simulink library "SUB_ECU_L4_MABX_HW_Interface_PIC_PB"  (R2018a)
settings: Solver=VariableStepAuto  StartTime=0.0  StopTime=10.0  RelTol=1e-3
PostLoadFcn:
  | , if any(exist('dsrtsu_mdlpostloadfcn', 'file') == [2, 3, 6]), try dsrtsu_mdlpostloadfcn('Execute', bdroot); catch fprintf('Error in PostLoadFcn (dsrtsu_mdlpostloadfcn) for model "%s":\n %s\n', bdroot, lasterr); end, end,
undefined symbols (not defined in the file or in its folder): CANR_PROPB_REAX_3_13_CHANNEL_APV, CANR_PROPB_REAX_4_13_CHANNEL_APV, CANR_PROPB_XPR_1_50_CHANNEL_APV, ENUM_CAN_RX_T, ENUM_CAN_TX_T, ENUM_REAX_OPERATION_MODE_T, ENUM_SIGNAL_HEALTH_T, ENUM_XBR_CONTROL_MODE_T, ENUM_XBR_EBI_MODE_T, ENUM_XBR_PASS_THROUGH_ACTIVE_T, ENUM_XBR_PRIORITY_T, ENUM_XPR_INHIBIT_PARK_MANUAL_T, ENUM_XPR_INHIBIT_UNPARK_MANUAL_T, ENUM_XPR_PARK_MANUAL_T, ENUM_XPR_UNPARK_MANUAL_T, PROPB_REAX_1_E4_DES_POS_SIG_SRC_APV, PROPB_REAX_1_E4_DESIRED_OPMODE_APV, PROPB_REAX_1_E4_DESIRED_POSITION_APV, PROPB_REAX_CHANNEL_APV, ptc_matlab_lib
libraries: PTC_MBDS_LIB x293, rtican x158, simulink x61, EmE_MBD_Blockset x38, rti1401lib_dio_type4 x14, simulink_need_slupdate x7, $bdroot x5, rti1401lib_adc_type4 x3, rtmapslib x3, dsa_tcpip_lib x2, SUB_ECU_L4_MABX_HW_Interface_PTC_1571 x1, rtitasklib x1
(part 5 of 49)

== system SUB_ECU_L4_MABX_HW_Interface_PIC_PB/ETHERNET/Data RX ==
  LinkStatus : Inport
  Status : Inport  Port=2
  SizeReceived : Inport  Port=3
  DataReceived : Inport  Port=4
  AND : Logic  IconShape=distinctive  AllPortsSameDT=off  OutDataTypeStr=boolean
  AND1 : Logic  IconShape=distinctive  AllPortsSameDT=off  OutDataTypeStr=boolean
  Bus Creator1 : BusCreator  Inputs=8
  Bus Selector2 : BusSelector  OutputSignals=rxNewData
  Bus Selector3 : BusSelector  OutputSignals=Heartbeat,SupervisorMode,CurrentAzimuth,TargetAzimuth,CurrentVelocity,TargetVelocity,Curvature,CrosstrackError,GPS_X,GPS_Y,GPS_Time
  Data Type Conversion : DataTypeConversion
  EQ : PTC_MBDS_LIB/MBDS Standard Library/Basic Operations/Logic and Bit Operations/EQ  InputSameDT=on  PTC_MBDS_BlockVersion=5.41  PTC_BlockType=PTC_MBDS_EQ
      settings: SourceProductName=PACCAR Technical Center MBDS Library
  Failure : Constant  Value=3  OutDataTypeStr=uint8
  No Data : Constant  Value=0  OutDataTypeStr=double
  RTMaps Health Check : Subsystem
  RTMapsDecode : rtmapslib/RTMapsDecode  paramBusName=RTMapsRX
      settings: AttributesFormatString=Bus: %<paramBusName>  SourceProductName=dSPACE RTMaps Interface Blockset
  Supervisor_Autonomous_Mode : Constant  Value=2  OutDataTypeStr=Inherit: Inherit via back propagation
  Switch{,1..9} (10 alike) : Switch  Criteria=u2 > Threshold
  Terminator{,1..4} (5 alike) : Terminator
  for_logging{,1..6} (7 alike) : Gain
  for_logging7 : Gain  OutDataTypeStr=int8
  m/s_to_km/h : Gain  Gain=3.6
  m/s_to_km/h_2 : Gain  Gain=3.6
  PIC_Bus : Outport
  wires:
  EQ/1 -> AND1/2
  AND1/1 -> Bus Creator1/1  "SystemsOk"
  Supervisor_Autonomous_Mode/1 -> EQ/1
  SizeReceived/1 -> Data Type Conversion/1
  DataReceived/1 -> RTMapsDecode/1
  Status/1 -> Bus Selector2/1
  Switch9/1 -> EQ/2, Bus Creator1/2  "SupervisorMode"
  Switch/1 -> Bus Creator1/3  "CurrentAzimuth_rad"
  for_logging2/1 -> Switch4/1
  Bus Selector2/1 -> RTMapsDecode/3  "<rxNewData>"
  Bus Selector3/2 -> for_logging7/1  "<SupervisorMode>"
  RTMaps Health Check/1(Status) -> AND/2  "RTMapsOk"
  AND/1 -> Switch/2, Switch1/2, Switch2/2, Switch3/2, Switch4/2, Switch5/2, Switch6/2, Switch7/2, Switch8/2, Switch9/2, AND1/1  "RTMapsOk"
  Bus Selector3/4 -> for_logging1/1  "<TargetAzimuth>"
  for_logging/1 -> Switch/1
  Switch3/1 -> Bus Creator1/6  "TargetVelocity_kph"
  Bus Selector3/1 -> RTMaps Health Check/1(Heartbeat)  "<Heartbeat>"
  Bus Selector3/7 -> for_logging2/1  "<Curvature>"
  Bus Selector3/9 -> for_logging4/1  "<GPS_X>"
  for_logging6/1 -> Switch8/1
  RTMapsDecode/3 -> Terminator2/1
  for_logging1/1 -> Switch1/1
  Bus Selector3/6 -> m/s_to_km/h_2/1  "<TargetVelocity>"
  RTMapsDecode/2 -> Terminator1/1
  Bus Selector3/3 -> for_logging/1  "<CurrentAzimuth>"
  Switch4/1 -> Bus Creator1/7  "Curvature"
  Bus Creator1/1 -> PIC_Bus/1  "PIC_Bus"
  Data Type Conversion/1 -> RTMapsDecode/2
  RTMapsDecode/1 -> Bus Selector3/1
  Switch6/1 -> Terminator/1  "GPS_X"
  Bus Selector3/5 -> m/s_to_km/h/1  "<CurrentVelocity>"
  Bus Selector3/8 -> for_logging3/1  "<CrosstrackError>"
  Bus Selector3/11 -> for_logging6/1  "<GPS_Time>"
  Bus Selector3/10 -> for_logging5/1  "<GPS_Y>"
  m/s_to_km/h/1 -> Switch2/1
  Switch1/1 -> Bus Creator1/4  "TargetAzimuth_rad"
  No Data/1 -> Switch4/3, Switch8/3, Switch7/3, Switch6/3, Switch5/3, Switch3/3, Switch2/3, Switch1/3, Switch/3
  Switch5/1 -> Bus Creator1/8  "CrosstrackError"
  for_logging4/1 -> Switch6/1
  for_logging3/1 -> Switch5/1
  LinkStatus/1 -> AND/1
  Switch8/1 -> Terminator4/1  "GPS_Time"
  m/s_to_km/h_2/1 -> Switch3/1
  for_logging7/1 -> Switch9/1  "SupervisorMode"
  for_logging5/1 -> Switch7/1
  Switch2/1 -> Bus Creator1/5  "CurrentVelocity_kph"
  Switch7/1 -> Terminator3/1  "GPS_Y"
  Failure/1 -> Switch9/3

== system SUB_ECU_L4_MABX_HW_Interface_PIC_PB/ETHERNET/Data TX ==
  In : Inport
  Bus Creator : BusCreator  Inputs=8  OutDataTypeStr=Bus: RTMapsTX  NonVirtualBus=on
  Bus Selector : BusSelector  OutputSignals=INPUTS.DIO_Bus.EStop,INPUTS.DIO_Bus.EnableSW,10msTask.AutonomousState.EngageReq,INPUTS.DIO_Bus.LogPB,10msTask.AutonomousState.AutonomousEnabled,10msTask.AutonomousState.MABX_Mode,INPUTS.DIO_Bus.BrakeSW
  Cast To Boolean : DataTypeConversion  OutDataTypeStr=boolean
  Heartbeat : DiscretePulseGenerator  Period=10  PulseWidth=5  SampleTime=0.01
  RTMapsEncode : rtmapslib/RTMapsEncode  TimestampMode=Simulation Time
      settings: SourceProductName=dSPACE RTMaps Interface Blockset
  SizeToSend : Outport
  DataToSend : Outport  Port=2
  wires:
  Bus Selector/7 -> Bus Creator/8  "<BrakeSW>"
  Bus Selector/4 -> Bus Creator/5  "<LogPB>"
  RTMapsEncode/2 -> SizeToSend/1
  RTMapsEncode/1 -> DataToSend/1
  Bus Creator/1 -> RTMapsEncode/1
  Cast To Boolean/1 -> Bus Creator/1  "MABX_Heartbeat"
  Heartbeat/1 -> Cast To Boolean/1
  In/1 -> Bus Selector/1
  Bus Selector/5 -> Bus Creator/6  "<AutonomousEnabled>"
  Bus Selector/6 -> Bus Creator/7  "<MABX_Mode>"
  Bus Selector/2 -> Bus Creator/3  "<EnableSW>"
  Bus Selector/1 -> Bus Creator/2  "<EStop>"
  Bus Selector/3 -> Bus Creator/4  "<EngageReq>"
